simulink model "three_phase_pwm_rectifier_voltage_regulated"  (R2015b)
settings: Solver=FixedStepAuto  SolverMode=SingleTasking  StartTime=0.0  StopTime=10.0  FixedStep=Ts  RelTol=1e-3
values from neighbouring files (symbols this model uses):
  Lline = 2e-4    (= 0.0002)    [three_phase_pwm_rectifier.m]
  Rline = 0.005    [three_phase_pwm_rectifier.m]
  Ts = 10e-6    (= 1e-05)    [three_phase_pwm_rectifier.m]
libraries: powerlib x25, powerlib_meascontrol x9, simulink x5
settings Model: Creator=Eren  LastModifiedBy=Eren

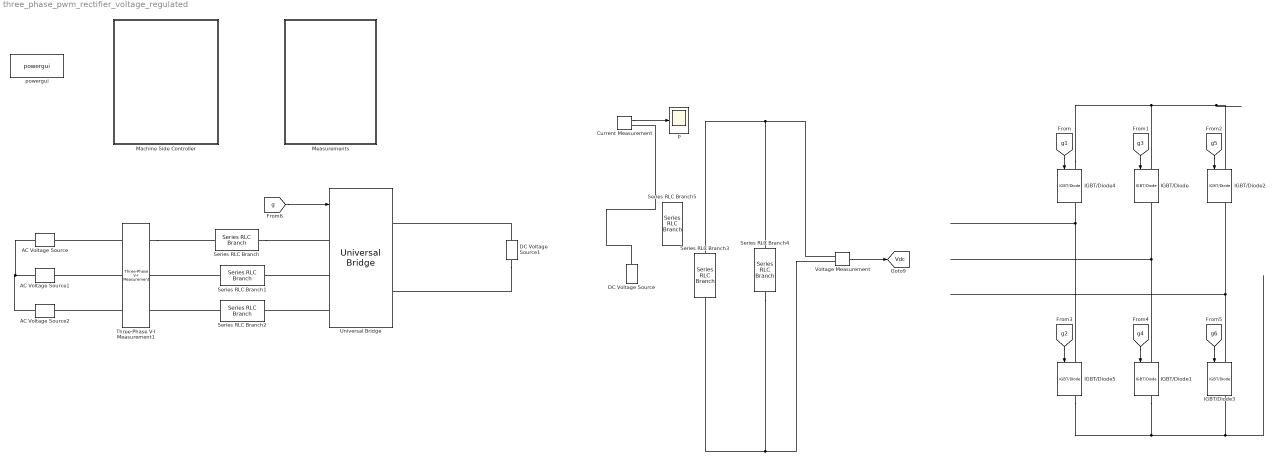
== system three_phase_pwm_rectifier_voltage_regulated ==
  AC Voltage Source : powerlib/Electrical Sources/AC Voltage Source  Amplitude=(690*sqrt(2))/sqrt(3)  Phase=0  Frequency=50  SampleTime=0  Measurements=Voltage  BusType=swing  Pref=10e3  Qref=0  Qmin=-inf  Qmax=+inf
  AC Voltage Source1 : powerlib/Electrical Sources/AC Voltage Source  Amplitude=(690*sqrt(2))/sqrt(3)  Phase=-120  Frequency=50  SampleTime=0  Measurements=Voltage  BusType=swing  Pref=10e3  Qref=0  Qmin=-inf  Qmax=+inf
  AC Voltage Source2 : powerlib/Electrical Sources/AC Voltage Source  Amplitude=(690*sqrt(2))/sqrt(3)  Phase=120  Frequency=50  SampleTime=0  Measurements=Voltage  BusType=swing  Pref=10e3  Qref=0  Qmin=-inf  Qmax=+inf
  Current Measurement : powerlib/Measurements/Current Measurement  PhasorSimulation=off  OutputType=Complex  PSBequivalent=0
  DC Voltage Source : powerlib/Electrical Sources/DC Voltage Source  Amplitude=1200  Measurements=None
  DC Voltage Source1 : powerlib/Electrical Sources/DC Voltage Source  Amplitude=1200  Measurements=None
  IGBT/Diode{,1..5} (6 alike) : powerlib/Power Electronics/IGBT//Diode  Ron=1e-3  Rs=1e5  Cs=inf  Measurements=on
  "Machine Side Controller " : Subsystem
  Measurements : Subsystem
  P : Scope
  Series RLC Branch : powerlib/Elements/Series RLC Branch  LConnTagsString=__new0  RConnTagsString=__new0  BranchType=RL  Resistance=Rline  Inductance=Lline  SetiL0=off  InitialCurrent=0  Capacitance=1e-6  Setx0=off  InitialVoltage=0  Measurements=None
  Series RLC Branch1 : powerlib/Elements/Series RLC Branch  LConnTagsString=__new0  RConnTagsString=__new0  BranchType=RL  Resistance=Rline  Inductance=Lline  SetiL0=off  InitialCurrent=0  Capacitance=1e-6  Setx0=off  InitialVoltage=0  Measurements=None
  Series RLC Branch2 : powerlib/Elements/Series RLC Branch  LConnTagsString=__new0  RConnTagsString=__new0  BranchType=RL  Resistance=Rline  Inductance=Lline  SetiL0=off  InitialCurrent=0  Capacitance=1e-6  Setx0=off  InitialVoltage=0  Measurements=None
  Series RLC Branch3 : powerlib/Elements/Series RLC Branch  LConnTagsString=__new0  RConnTagsString=__new0  BranchType=C  Resistance=1  Inductance=1e-3  SetiL0=off  InitialCurrent=0  Capacitance=2700e-6  Setx0=on  InitialVoltage=1200  Measurements=None
  Series RLC Branch4 : powerlib/Elements/Series RLC Branch  LConnTagsString=__new0  RConnTagsString=__new0  BranchType=R  Resistance=(1200)^2/2.75e6  Inductance=1e-3  SetiL0=off  InitialCurrent=0  Capacitance=1e-6  Setx0=off  InitialVoltage=0  Measurements=None
  Series RLC Branch5 : powerlib/Elements/Series RLC Branch  LConnTagsString=__new0  RConnTagsString=__new0  BranchType=R  Resistance=(1200)^2/2.75e6  Inductance=1e-3  SetiL0=off  InitialCurrent=0  Capacitance=1e-6  Setx0=off  InitialVoltage=0  Measurements=None
  Three-Phase V-I Measurement1 : powerlib/Measurements/Three-Phase V-I Measurement  VoltageMeasurement=phase-to-phase  SetLabelV=on  LabelV=Vsabc  Vpu=off  VpuLL=on  CurrentMeasurement=yes  SetLabelI=on  LabelI=Isabc  Ipu=on  Pbase=2.75e6  Vbase=690  OutputType=Complex  PhasorSimulation=off  PSBequivalent=0
  Universal Bridge : powerlib/Power Electronics/Universal Bridge  Arms=3  SnubberResistance=1e5  SnubberCapacitance=inf  Device=IGBT / Diodes  Ron=1e-3  Lon=0  ForwardVoltages="[  0  0  ]"  ForwardVoltage=0  GTOparameters=[ 10e-6 , 20e-6 ]  IGBTparameters=[ 1e-6 , 2e-6 ]  Measurements=None  Measurements_2=None  converterType=Rectifier
  Voltage Measurement : powerlib/Measurements/Voltage Measurement  PhasorSimulation=off  OutputType=Complex  PSBequivalent=0
  powergui : powerlib/powergui  Priority=2  SimulationMode=Discrete  SolverType=Tustin  SampleTime=Ts  frequency=60  SPID=off  DisableSnubberDevices=off  DisableRonSwitches=off  DisableVfSwitches=off  SwTol=0  DisplayEquations=off  Interpol=off  ExternalGateDelay=off  methode=off  Ts=0  FunctionMessages=off  echomessages=off  HookPort=off  EnableUseOfTLC=off  x0status=blocks  frequencyindice=0  Pbase=100e6  ErrMax=1e-4  Iterations=50  UnitsV=kV  UnitsW=MW  buscounter=0  RestoreLinks=warning  ResistiveCurrentMeasurement=off  Frange=[0:2:500]  Ylog=off  Xlog=on  ShowGrid=off  save=off  variable=ZData  structure=0  ZoomFFT=on  StartTime=0.0  cycles=1  DisplayStyle=1  fundamental=60  FreqAxis=off  MaxFrequency=1000  frequencyindicesteady=1  RmsSteady=1  display=off
  tag scope: Vdc=global
  wires:
  Voltage Measurement/1 -> [Vdc]
  Current Measurement/1 -> P/1
  [g1] -> IGBT/Diode4/1
  [g3] -> IGBT/Diode/1
  [g5] -> IGBT/Diode2/1
  [g2] -> IGBT/Diode5/1
  [g4] -> IGBT/Diode1/1
  [g6] -> IGBT/Diode3/1
  [g] -> Universal Bridge/1
  connections:
  AC Voltage Source2/LConn1 -- AC Voltage Source/LConn1 -- AC Voltage Source1/LConn1
  Series RLC Branch4/LConn1 -- Voltage Measurement/LConn1 -- Series RLC Branch3/LConn1
  Voltage Measurement/LConn2 -- Series RLC Branch3/RConn1 -- Series RLC Branch4/RConn1
  DC Voltage Source/RConn1 -- Current Measurement/RConn1
  IGBT/Diode4/RConn1 -- IGBT/Diode5/LConn1
  IGBT/Diode/RConn1 -- IGBT/Diode1/LConn1
  IGBT/Diode2/RConn1 -- IGBT/Diode3/LConn1
  IGBT/Diode4/LConn1 -- IGBT/Diode/LConn1 -- IGBT/Diode2/LConn1
  IGBT/Diode3/RConn1 -- IGBT/Diode5/RConn1 -- IGBT/Diode1/RConn1
  DC Voltage Source1/RConn1 -- Universal Bridge/RConn1
  DC Voltage Source1/LConn1 -- Universal Bridge/RConn2
  Three-Phase V-I Measurement1/LConn1 -- AC Voltage Source/RConn1
  Three-Phase V-I Measurement1/RConn1 -- Series RLC Branch/LConn1
  Three-Phase V-I Measurement1/LConn2 -- AC Voltage Source1/RConn1
  Three-Phase V-I Measurement1/LConn3 -- AC Voltage Source2/RConn1
  Series RLC Branch1/LConn1 -- Three-Phase V-I Measurement1/RConn2
  Series RLC Branch2/LConn1 -- Three-Phase V-I Measurement1/RConn3
  Series RLC Branch/RConn1 -- Universal Bridge/LConn1
  Universal Bridge/LConn2 -- Series RLC Branch1/RConn1
  Universal Bridge/LConn3 -- Series RLC Branch2/RConn1

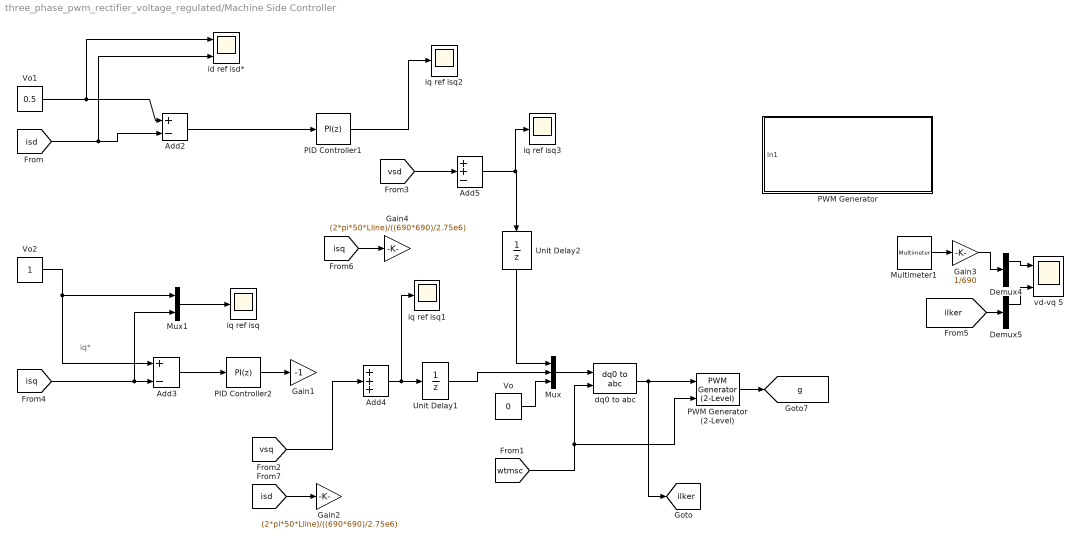
== system three_phase_pwm_rectifier_voltage_regulated/Machine Side Controller  ==
  note: iq*
  Add2 : Sum  Inputs=+-
  Add3 : Sum  Inputs=+-
  Add4 : Sum  Inputs=+++
  Add5 : Sum  Inputs=++-
  Demux4 : Demux  Outputs=3
  Demux5 : Demux  Outputs=3
  Gain1 : Gain  Gain=-1
  Gain2 : Gain  Gain=(2*pi*50*Lline)/((690*690)/2.75e6)
  Gain3 : Gain  Gain=1/690
  Gain4 : Gain  Gain=(2*pi*50*Lline)/((690*690)/2.75e6)
  Multimeter1 : powerlib/Measurements/Multimeter  PhasorSimulation=off  OutputType=Complex  sel=[3 2 1]  L=3  Gain=[1 1 1]  yselected={'Usrc: AC Voltage Source','Usrc: AC Voltage Source1','Usrc: AC Voltage Source2'};  PSBOutputType=1  PSBequivalent=0  AxesSetting=[0,0.1,-100,100]  Display=0  SavedBlockNames=-11
  Mux : Mux  Inputs=3
  Mux1 : Mux  Inputs=2
  PID Controller1 : simulink/Continuous/PID Controller  Controller=PI  TimeDomain=Discrete-time  SampleTime=Ts  IntegratorMethod=Forward Euler  FilterMethod=Forward Euler  Form=Parallel  UseFilter=on  ControllerParametersSource=internal  P=0.1  I=0.01  D=0  N=100  InitialConditionSource=internal  InitialConditionForIntegrator=0  InitialConditionForFilter=0  ExternalReset=none  LimitOutput=on  UpperSaturationLimit=1.5  LowerSaturationLimit=-1.5  LinearizeAsGain=on  AntiWindupMode=none  Kb=1  TrackingMode=off  Kt=1  PParamMin=[]  PParamMax=[]  IParamMin=[]  IParamMax=[]  DParamMin=[]  DParamMax=[]  NParamMin=[]  NParamMax=[]  KbParamMin=[]  KbParamMax=[]  KtParamMin=[]  KtParamMax=[]  POutMin=[]  POutMax=[]  IOutMin=[]  IOutMax=[]  DOutMin=[]  DOutMax=[]  NOutMin=[]  NOutMax=[]  KbOutMin=[]  KbOutMax=[]  KtOutMin=[]  KtOutMax=[]  IntegratorOutMin=[]  IntegratorOutMax=[]  FilterOutMin=[]  FilterOutMax=[]  SumOutMin=[]  SumOutMax=[]  SumI1OutMin=[]  SumI1OutMax=[]  SumI2OutMin=[]  SumI2OutMax=[]  SumI3OutMin=[]  SumI3OutMax=[]  SumDOutMin=[]  SumDOutMax=[]  SaturationOutMin=[]  SaturationOutMax=[]  IntegratorContinuousStateAttributes=''  IntegratorStateMustResolveToSignalObject=off  IntegratorRTWStateStorageClass=Auto  FilterContinuousStateAttributes=''  FilterStateMustResolveToSignalObject=off  FilterRTWStateStorageClass=Auto  DifferentiatorICPrevScaledInput=0  DifferentiatorOutMin=[]  DifferentiatorOutMax=[]
  PID Controller2 : simulink/Continuous/PID Controller  Controller=PI  TimeDomain=Discrete-time  SampleTime=Ts  IntegratorMethod=Forward Euler  FilterMethod=Forward Euler  Form=Parallel  UseFilter=on  ControllerParametersSource=internal  P=0.1  I=0.01  D=0  N=100  InitialConditionSource=internal  InitialConditionForIntegrator=0  InitialConditionForFilter=0  ExternalReset=none  LimitOutput=on  UpperSaturationLimit=2  LowerSaturationLimit=-2  LinearizeAsGain=on  AntiWindupMode=none  Kb=1  TrackingMode=off  Kt=1  PParamMin=[]  PParamMax=[]  IParamMin=[]  IParamMax=[]  DParamMin=[]  DParamMax=[]  NParamMin=[]  NParamMax=[]  KbParamMin=[]  KbParamMax=[]  KtParamMin=[]  KtParamMax=[]  POutMin=[]  POutMax=[]  IOutMin=[]  IOutMax=[]  DOutMin=[]  DOutMax=[]  NOutMin=[]  NOutMax=[]  KbOutMin=[]  KbOutMax=[]  KtOutMin=[]  KtOutMax=[]  IntegratorOutMin=[]  IntegratorOutMax=[]  FilterOutMin=[]  FilterOutMax=[]  SumOutMin=[]  SumOutMax=[]  SumI1OutMin=[]  SumI1OutMax=[]  SumI2OutMin=[]  SumI2OutMax=[]  SumI3OutMin=[]  SumI3OutMax=[]  SumDOutMin=[]  SumDOutMax=[]  SaturationOutMin=[]  SaturationOutMax=[]  IntegratorContinuousStateAttributes=''  IntegratorStateMustResolveToSignalObject=off  IntegratorRTWStateStorageClass=Auto  FilterContinuousStateAttributes=''  FilterStateMustResolveToSignalObject=off  FilterRTWStateStorageClass=Auto  DifferentiatorICPrevScaledInput=0  DifferentiatorOutMin=[]  DifferentiatorOutMax=[]
  "PWM Generator " : Subsystem
  PWM Generator (2-Level) : powerlib_meascontrol/Pulse & Signal Generators/PWM Generator (2-Level)  ModulatorType=Three-phase bridge (6 pulses)  ModulatorMode=Synchronized  Fc=drivefreq  Pc=90  nF=60  MinMax="[ -1  1 ]"  SamplingTechnique=Natural  ModulatingSignals=off  m=0.8  Freq=60  Phase=0  Ts=Ts  ShowCarrierOutport=off
  Unit Delay1 : UnitDelay  SampleTime=Ts
  Unit Delay2 : UnitDelay  SampleTime=Ts
  Vo : Constant  Value=0
  Vo1 : Constant  Value=0.5
  Vo2 : Constant
  dq0 to abc : powerlib_meascontrol/Transformations/dq0 to abc  Alignment=90 degrees behind phase A axis
  id ref isd* : Scope  NumInputPorts=2
  iq ref isq{,1..3} (4 alike) : Scope
  vd-vq 5 : Scope  NumInputPorts=2
  tag scope: g=global, ilker=global
  wires:
  Mux/1 -> dq0 to abc/1
  Vo1/1 -> id ref isd*/1, Add2/1
  Vo/1 -> Mux/3
  [isq] -> Mux1/2, Add3/2
  Add3/1 -> PID Controller2/1
  Add2/1 -> PID Controller1/1
  [isd] -> id ref isd*/2, Add2/2
  Mux1/1 -> iq ref isq/1
  PID Controller2/1 -> Gain1/1
  dq0 to abc/1 -> PWM Generator (2-Level)/1, [ilker]
  [wtmsc] -> PWM Generator (2-Level)/2, dq0 to abc/2
  Vo2/1 -> Add3/1, Mux1/1
  [vsq] -> Add4/2
  [vsd] -> Add5/2
  Add5/1 -> iq ref isq3/1, Unit Delay2/1
  Add4/1 -> Unit Delay1/1, iq ref isq1/1
  PWM Generator (2-Level)/1 -> [g]
  Unit Delay1/1 -> Mux/2
  Unit Delay2/1 -> Mux/1
  Multimeter1/1 -> Gain3/1
  [ilker] -> Demux5/1
  Gain3/1 -> Demux4/1
  Demux4/1 -> vd-vq 5/1
  Demux5/1 -> vd-vq 5/2
  PID Controller1/1 -> iq ref isq2/1
  [isd] -> Gain2/1
  [isq] -> Gain4/1

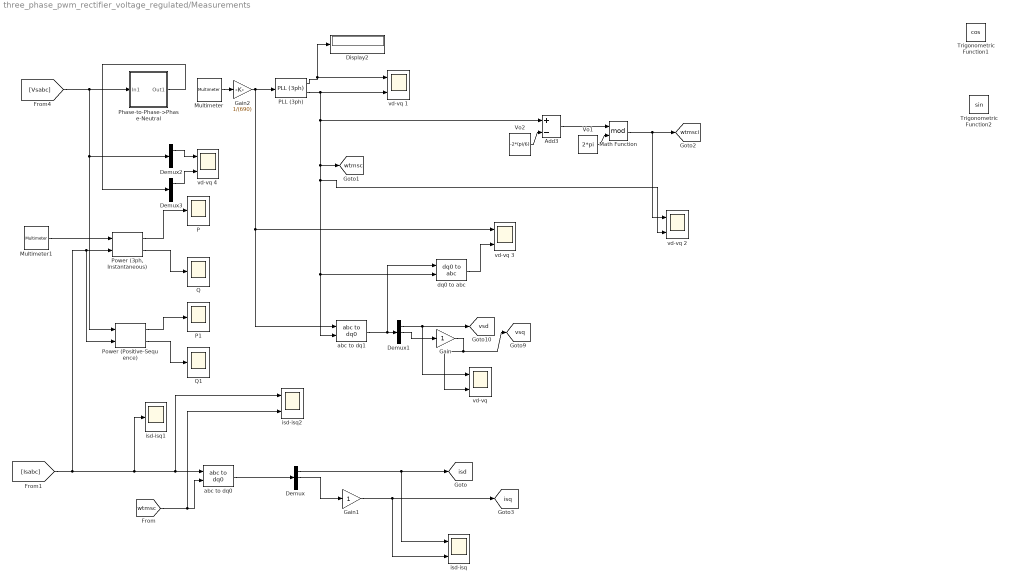
== system three_phase_pwm_rectifier_voltage_regulated/Measurements ==
  Add3 : Sum  Inputs=+-
  Demux{,1..3} (4 alike) : Demux  Outputs=3
  Display2 : Display
  Gain : Gain
  Gain1 : Gain
  Gain2 : Gain  Gain=1/(690)
  Math Function : Math  Operator=mod  SaturateOnIntegerOverflow=on
  Multimeter : powerlib/Measurements/Multimeter  PhasorSimulation=off  OutputType=Complex  sel=[3 2 1]  L=3  Gain=[1 1 1]  yselected={'Usrc: AC Voltage Source','Usrc: AC Voltage Source1','Usrc: AC Voltage Source2'};  PSBOutputType=1  PSBequivalent=0  AxesSetting=[0,0.1,-100,100]  Display=0  SavedBlockNames=-11
  Multimeter1 : powerlib/Measurements/Multimeter  PhasorSimulation=off  OutputType=Complex  sel=[3 2 1]  L=3  Gain=[1 1 1]  yselected={'Usrc: AC Voltage Source','Usrc: AC Voltage Source1','Usrc: AC Voltage Source2'};  PSBOutputType=1  PSBequivalent=0  AxesSetting=[0,0.1,-100,100]  Display=0  SavedBlockNames=-11
  P : Scope
  P1 : Scope
  PLL (3ph) : powerlib_meascontrol/PLL/PLL (3ph)  Fmin=45  Par_Init=[0, 50]  ParK=[180, 3200, 1]  TcD=1e-4  MaxRateChangeFreq=12  FilterCutOffFreq=25  Ts=0  AGC=on
  Phase-to-Phase->Phase-Neutral : Subsystem
  "Power (3ph, Instantaneous)" : powerlib_meascontrol/Measurements/Power (3ph, Instantaneous)
  Power (Positive-Sequence) : powerlib_meascontrol/Measurements/Power (Positive-Sequence)  Freq=60  Vinit=[0, 0]  Iinit=[0, 0]  Ts=0
  Q : Scope
  Q1 : Scope
  Trigonometric Function1 : Trigonometry  Operator=cos
  Trigonometric Function2 : Trigonometry
  Vo1 : Constant  Value=2*pi
  Vo2 : Constant  Value=-2*(pi/6)
  abc to dq0 : powerlib_meascontrol/Transformations/abc to dq0  Alignment=90 degrees behind phase A axis
  abc to dq1 : powerlib_meascontrol/Transformations/abc to dq0  Alignment=Aligned with phase A axis
  dq0 to abc : powerlib_meascontrol/Transformations/dq0 to abc  Alignment=Aligned with phase A axis
  isd-isq : Scope  NumInputPorts=2
  isd-isq1 : Scope
  isd-isq2 : Scope  NumInputPorts=2
  vd-vq {,1..4} (5 alike) : Scope  NumInputPorts=2
  tag scope: isd=global, isq=global, vsd=global, vsq=global, wtmsc=global, wtmsci=global
  wires:
  [Vsabc] -> Power (Positive-Sequence)/1, Demux2/1, Phase-to-Phase->Phase-Neutral/1(In1)
  PLL (3ph)/1 -> Display2/1, vd-vq 1/1
  [Isabc] -> Power (Positive-Sequence)/2, "Power (3ph, Instantaneous)"/2, isd-isq1/1, isd-isq2/1, abc to dq0/1
  abc to dq0/1 -> Demux/1
  abc to dq1/1 -> dq0 to abc/1, Demux1/1
  Demux1/1 -> "vd-vq "/1, [vsd]
  Demux1/2 -> Gain/1
  Demux/1 -> isd-isq/1, [isd]
  Demux/2 -> Gain1/1
  Math Function/1 -> vd-vq 2/1, [wtmsci]
  Add3/1 -> Math Function/1
  Vo2/1 -> Add3/2
  Vo1/1 -> Math Function/2
  [wtmsc] -> isd-isq2/2, abc to dq0/2
  PLL (3ph)/2 -> Add3/1, [wtmsc], vd-vq 2/2, dq0 to abc/2, abc to dq1/2, vd-vq 1/2
  "Power (3ph, Instantaneous)"/1 -> P/1
  "Power (3ph, Instantaneous)"/2 -> Q/1
  Power (Positive-Sequence)/1 -> P1/1
  Power (Positive-Sequence)/2 -> Q1/1
  Gain/1 -> "vd-vq "/2, [vsq]
  Gain1/1 -> [isq], isd-isq/2
  dq0 to abc/1 -> vd-vq 3/2
  Phase-to-Phase->Phase-Neutral/1(Out1) -> Demux3/1
  Demux3/1 -> vd-vq 4/2
  Demux2/1 -> vd-vq 4/1
  Multimeter/1 -> Gain2/1
  Gain2/1 -> vd-vq 3/1, abc to dq1/1, PLL (3ph)/1
  Multimeter1/1 -> "Power (3ph, Instantaneous)"/1

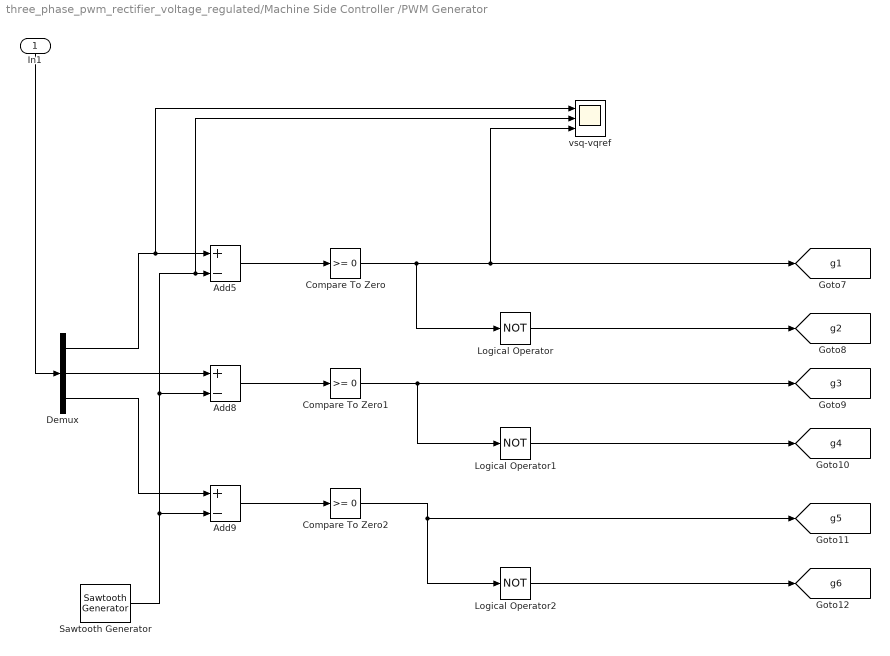
== system three_phase_pwm_rectifier_voltage_regulated/Machine Side Controller /PWM Generator  ==
  In1 : Inport
  Add5 : Sum  Inputs=+-
  Add8 : Sum  Inputs=+-
  Add9 : Sum  Inputs=+-
  Compare To Zero : simulink/Logic and Bit Operations/Compare To Zero  relop=>=  OutDataTypeStr=boolean
  Compare To Zero1 : simulink/Logic and Bit Operations/Compare To Zero  relop=>=  OutDataTypeStr=boolean
  Compare To Zero2 : simulink/Logic and Bit Operations/Compare To Zero  relop=>=  OutDataTypeStr=boolean
  Demux : Demux  Outputs=3
  Logical Operator : Logic  Operator=NOT  AllPortsSameDT=off  OutDataTypeStr=boolean
  Logical Operator1 : Logic  Operator=NOT  AllPortsSameDT=off  OutDataTypeStr=boolean
  Logical Operator2 : Logic  Operator=NOT  AllPortsSameDT=off  OutDataTypeStr=boolean
  Sawtooth Generator : powerlib_meascontrol/Pulse & Signal Generators/Sawtooth Generator  Freq=drivefreq  Phase=0  Ts=Ts
  vsq-vqref : Scope  NumInputPorts=3
  tag scope: g1=global, g2=global, g3=global, g4=global, g5=global, g6=global
  wires:
  Add8/1 -> Compare To Zero1/1
  Demux/1 -> vsq-vqref/1, Add5/1
  Compare To Zero/1 -> Logical Operator/1, [g1], vsq-vqref/3
  Add9/1 -> Compare To Zero2/1
  Demux/2 -> Add8/1
  Demux/3 -> Add9/1
  Logical Operator2/1 -> [g6]
  Add5/1 -> Compare To Zero/1
  In1/1 -> Demux/1
  Sawtooth Generator/1 -> Add8/2, vsq-vqref/2, Add5/2, Add9/2
  Compare To Zero1/1 -> [g3], Logical Operator1/1
  Logical Operator/1 -> [g2]
  Compare To Zero2/1 -> [g5], Logical Operator2/1
  Logical Operator1/1 -> [g4]

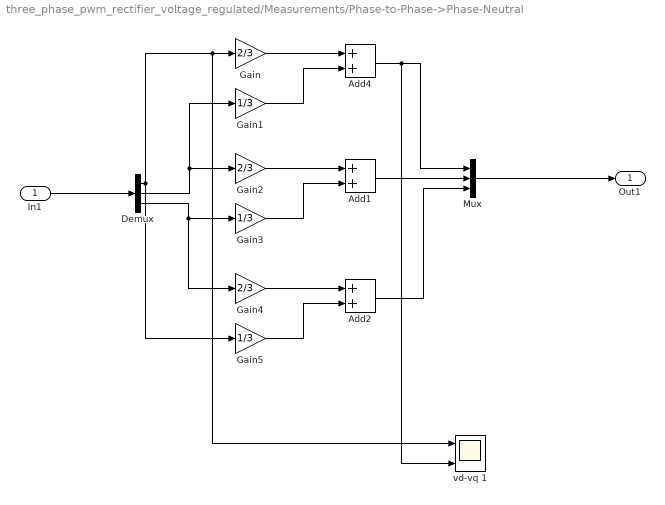
== system three_phase_pwm_rectifier_voltage_regulated/Measurements/Phase-to-Phase->Phase-Neutral ==
  In1 : Inport
  Add1 : Sum
  Add2 : Sum
  Add4 : Sum
  Demux : Demux  Outputs=3
  Gain : Gain  Gain=2/3
  Gain1 : Gain  Gain=1/3
  Gain2 : Gain  Gain=2/3
  Gain3 : Gain  Gain=1/3
  Gain4 : Gain  Gain=2/3
  Gain5 : Gain  Gain=1/3
  Mux : Mux  Inputs=3
  vd-vq 1 : Scope  NumInputPorts=2
  Out1 : Outport
  wires:
  Add1/1 -> Mux/2
  Gain/1 -> Add4/1
  Gain1/1 -> Add4/2
  Gain5/1 -> Add2/2
  Gain4/1 -> Add2/1
  Demux/1 -> vd-vq 1/1, Gain/1, Gain5/1
  In1/1 -> Demux/1
  Gain3/1 -> Add1/2
  Gain2/1 -> Add1/1
  Demux/2 -> Gain1/1, Gain2/1
  Demux/3 -> Gain4/1, Gain3/1
  Add2/1 -> Mux/3
  Add4/1 -> vd-vq 1/2, Mux/1
  Mux/1 -> Out1/1
